simulink model "Resonant"  (R2022b)
settings: Solver=VariableStepAuto  StartTime=0.0  StopTime=50  RelTol=1e-3
settings Model: Creator=tolen  LastModifiedBy=tolen

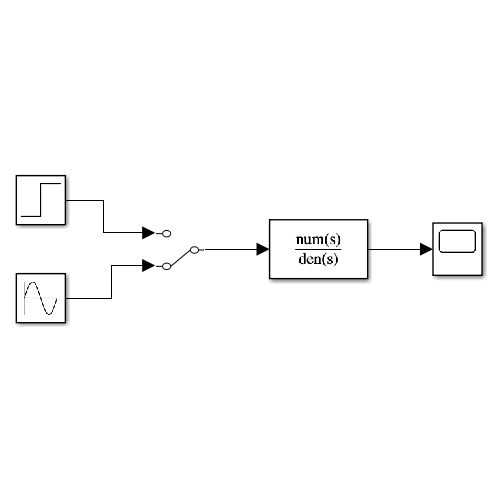
[thumbnail: Simulink's stored preview of the top-level diagram]
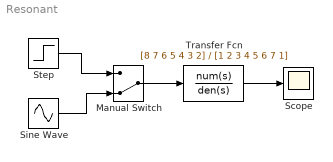
== system Resonant ==
  Manual Switch : ManualSwitch  CurrentSetting=0
  Scope : Scope
  Sine Wave : Sin  SampleTime=0
  Step : Step  Time=0  SampleTime=0
  Transfer Fcn : TransferFcn  Numerator=[8 7 6 5 4 3 2]  Denominator=[1 2 3 4 5 6 7 1]
  wires:
  Manual Switch/1 -> Transfer Fcn/1
  Transfer Fcn/1 -> Scope/1
  Step/1 -> Manual Switch/1
  Sine Wave/1 -> Manual Switch/2
